simulink model "idiot_TF"  (R2022b)
settings: Solver=VariableStepAuto  StartTime=0.0  StopTime=10.0  RelTol=1e-3
settings Model: Creator=yeyi5  LastModifiedBy=yeyi5

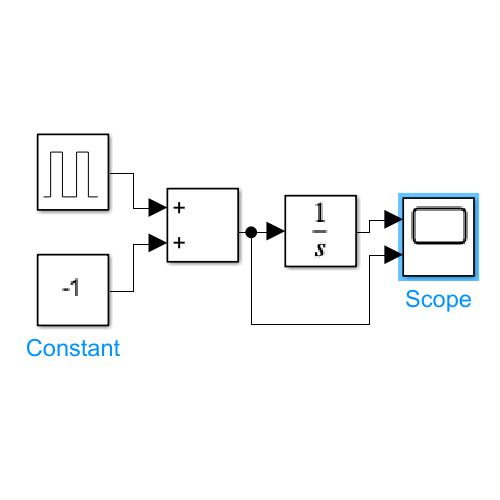
[thumbnail: Simulink's stored preview of the top-level diagram]
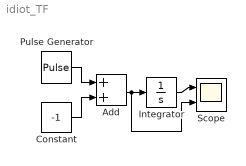
== system idiot_TF ==
  Add : Sum
  Constant : Constant  Value=-1
  Integrator : Integrator
  Pulse Generator : DiscretePulseGenerator  PulseType=Time based  Amplitude=2  PulseWidth=50
  Scope : Scope  NumInputPorts=2
  wires:
  Pulse Generator/1 -> Add/1
  Constant/1 -> Add/2
  Add/1 -> Scope/2, Integrator/1
  Integrator/1 -> Scope/1
